simulink model "helico_model_kne24"  (R2017a)
settings: Solver=FixedStepAuto  StartTime=0.0  StopTime=par.tend  FixedStep=par.ts  MaxStep=1e-3  RelTol=1e-3
values from neighbouring files (symbols this model uses):
  N = 4001    [workspace.mat]
  par =     [workspace.mat]
  par_id = struct    [model_benchmark_init.m]    (also in workspace.mat = )
undefined symbols (not defined in the file or in its folder): X, Y, Z
libraries: sm_lib x25, nesl_utility x11, simulink x1
settings Model: Creator=mirko  LastModifiedBy=obrusvit

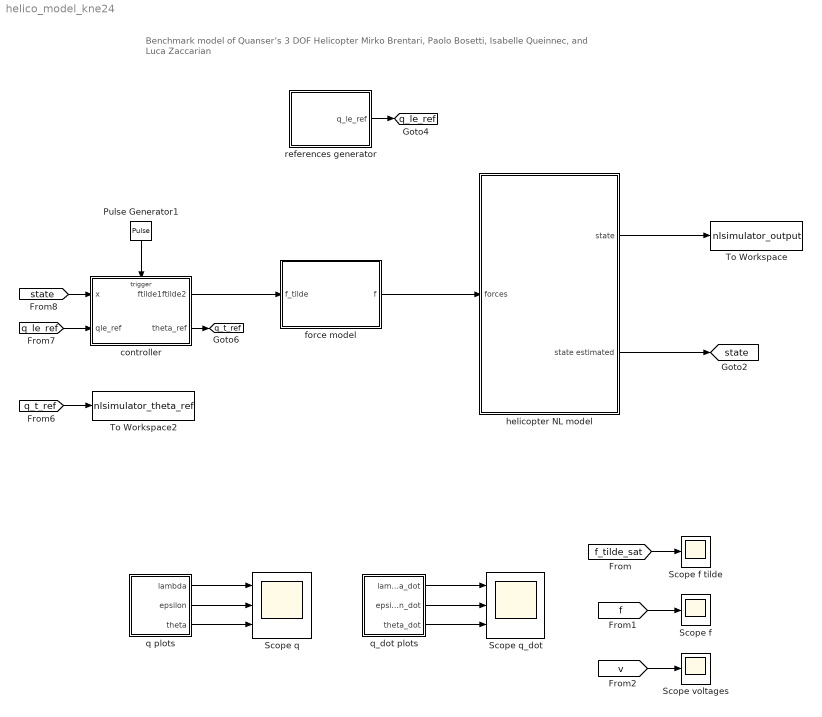
== system helico_model_kne24 ==
  note: Benchmark model of Quanser’s 3 DOF Helicopter
      | Mirko Brentari, Paolo Bosetti, Isabelle Queinnec, and Luca Zaccarian
  Pulse Generator1 : DiscretePulseGenerator  PulseType=Time based  Period=0.01  PulseWidth=50
  Scope f : Scope
  Scope f tilde : Scope
  Scope q : Scope  NumInputPorts=3
  Scope q_dot : Scope  NumInputPorts=3
  Scope voltages : Scope
  To Workspace : ToWorkspace  VariableName=nlsimulator_output  SaveFormat=Timeseries  SampleTime=-1
  To Workspace2 : ToWorkspace  VariableName=nlsimulator_theta_ref  SaveFormat=Timeseries  SampleTime=-1
  controller : Subsystem
  force model : Subsystem
  helicopter NL model : Subsystem
  q plots : Subsystem
  q_dot plots : Subsystem
  references generator : Subsystem
  tag scope: q_le_ref=global, q_t_ref=global, state=global
  wires:
  helicopter NL model/1(state) -> To Workspace/1
  references generator/1(q_le_ref) -> [q_le_ref]
  q plots/2(epsilon) -> Scope q/2
  q plots/1(lambda) -> Scope q/1
  q_dot plots/1(lambda_dot) -> Scope q_dot/1
  q plots/3(theta) -> Scope q/3
  q_dot plots/3(theta_dot) -> Scope q_dot/3
  q_dot plots/2(epsilon_dot) -> Scope q_dot/2
  helicopter NL model/2(state estimated) -> [state]
  [q_t_ref] -> To Workspace2/1
  Pulse Generator1/1 -> controller/Trigger
  controller/2(theta_ref) -> [q_t_ref]
  [state] -> controller/1(x)
  [q_le_ref] -> controller/2(qle_ref)
  controller/1(ftilde1ftilde2) -> force model/1(f_tilde)
  force model/1(f) -> helicopter NL model/1(forces)
  [f] -> Scope f/1
  [f_tilde_sat] -> Scope f tilde/1
  [v] -> Scope voltages/1

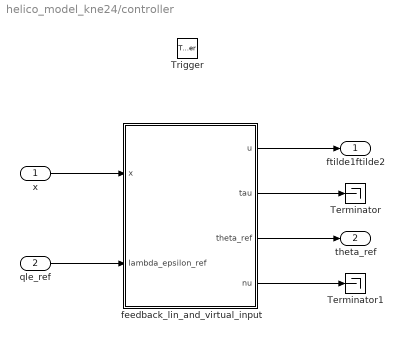
== system helico_model_kne24/controller ==
  x : Inport
  qle_ref : Inport  Port=2
  Trigger : TriggerPort  VariantControl=Variant  PortDimensions=1
  Terminator : Terminator
  Terminator1 : Terminator
  feedback_lin_and_virtual_input : MATLAB Function  TreatAsAtomicUnit=on
  ftilde1ftilde2 : Outport
  theta_ref : Outport  Port=2
  wires:
  qle_ref/1 -> feedback_lin_and_virtual_input/2(lambda_epsilon_ref)
  feedback_lin_and_virtual_input/3(theta_ref) -> theta_ref/1
  feedback_lin_and_virtual_input/2(tau) -> Terminator/1
  feedback_lin_and_virtual_input/1(u) -> ftilde1ftilde2/1
  x/1 -> feedback_lin_and_virtual_input/1(x)
  feedback_lin_and_virtual_input/4(nu) -> Terminator1/1

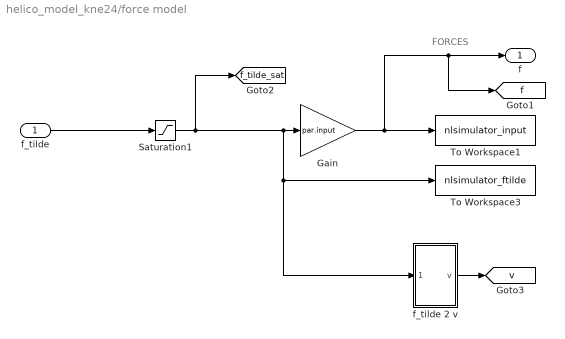
== system helico_model_kne24/force model ==
  note: FORCES
  f_tilde : Inport
  Gain : Gain  Gain=par.input
  Saturation1 : Saturate  UpperLimit=1  LowerLimit=-0.23
  To Workspace1 : ToWorkspace  VariableName=nlsimulator_input  SaveFormat=Timeseries  SampleTime=par.ts
  To Workspace3 : ToWorkspace  VariableName=nlsimulator_ftilde  SaveFormat=Timeseries  SampleTime=par.ts
  f_tilde 2 v : Subsystem
  f : Outport
  tag scope: f=global, f_tilde_sat=global, v=global
  wires:
  Saturation1/1 -> [f_tilde_sat], f_tilde 2 v/1(f_tilde), To Workspace3/1, Gain/1
  f_tilde/1 -> Saturation1/1
  Gain/1 -> [f], f/1, To Workspace1/1
  f_tilde 2 v/1(v) -> [v]

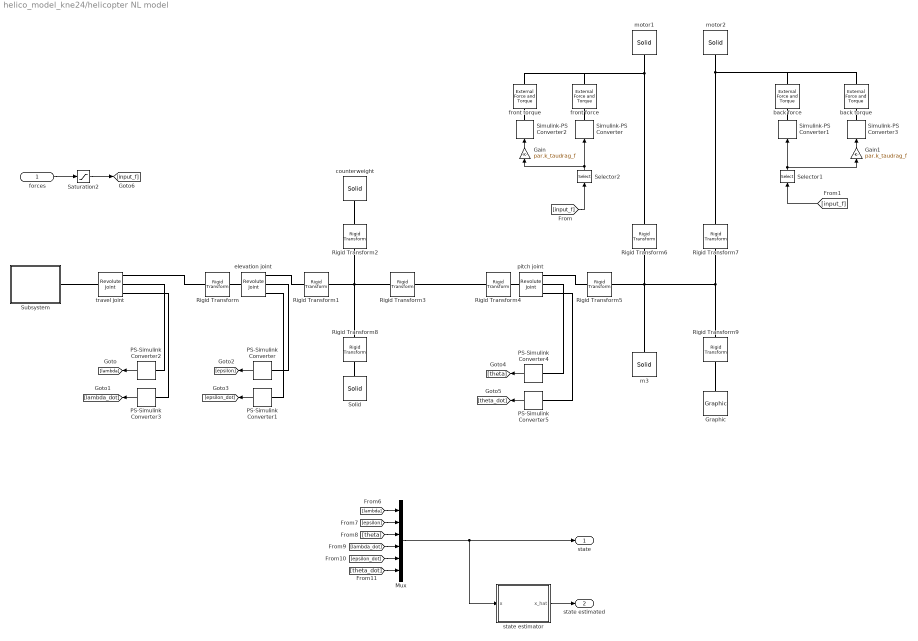
== system helico_model_kne24/helicopter NL model ==
  forces : Inport
  Gain : Gain  Gain=par.k_taudrag_f
  Gain1 : Gain  Gain=par.k_taudrag_f
  Graphic : sm_lib/Body Elements/Graphic  GraphicType=Marker  MarkerShape=Sphere  MarkerSize=10  GraphicVisPropType=SimpleVisualProperties  GraphicDiffuseColor=[1.0 0.0 0.2]  GraphicSpecularColor=[0.5 0.5 0.5 1.0]  GraphicAmbientColor=[0.15 0.15 0.15 1.0]  GraphicEmissiveColor=[0.0 0.0 0.0 1.0]  GraphicShininess=75  GraphicOpacity=0.5
      settings: SourceProductName=Simscape Multibody
  Mux : Mux  Inputs=6
  PS-Simulink Converter{,1..5} (6 alike) : nesl_utility/PS-Simulink Converter  PhysicalDomain=network_engine_domain  SubClassName=ps_output  LeftPortType=input  RightPortType=output  PseudoPeriodic=off  Frequencies=[]  Unit=1  AffineConversion=off
  Rigid Transform : sm_lib/Frames and Transforms/Rigid Transform  TranslationMethod=None  TranslationStandardOffset=0  TranslationLengthUnit=m  TranslationStandardAxis=+Z  TranslationCartesianOffset=[0 0 0]  TranslationROffset=0  TranslationROffsetUnits=m  TranslationZOffset=0  TranslationZOffsetUnits=m  TranslationThetaOffset=0  TranslationThetaOffsetUnits=deg  RotationMethod=StandardAxis  RotationAngleUnits=deg  RotationStandardAxis=+X  RotationAngle=90  RotationArbitraryAxis=[0 0 1]  FollAlignAxisA=+Z  BaseAlignAxisA=+Y  FollAlignAxisB=+X  BaseAlignAxisB=+X  RotationSequenceAxes=FollowerAxes  RotationSequence=XYX  RotationSequenceAngles=[0 0 0]  RotationSequenceAnglesUnits=deg  RotationMatrix=[1 0 0; 0 1 0; 0 0 1]
  Rigid Transform1 : sm_lib/Frames and Transforms/Rigid Transform  TranslationMethod=None  TranslationStandardOffset=0  TranslationLengthUnit=m  TranslationStandardAxis=+Z  TranslationCartesianOffset=[1 0 0]  TranslationROffset=0  TranslationROffsetUnits=m  TranslationZOffset=0  TranslationZOffsetUnits=m  TranslationThetaOffset=0  TranslationThetaOffsetUnits=deg  RotationMethod=StandardAxis  RotationAngleUnits=deg  RotationStandardAxis=+X  RotationAngle=-90  RotationArbitraryAxis=[0 0 1]  FollAlignAxisA=+Z  BaseAlignAxisA=+Y  FollAlignAxisB=+X  BaseAlignAxisB=+X  RotationSequenceAxes=FollowerAxes  RotationSequence=XYX  RotationSequenceAngles=[0 0 0]  RotationSequenceAnglesUnits=deg  RotationMatrix=[1 0 0; 0 1 0; 0 0 1]
  Rigid Transform2 : sm_lib/Frames and Transforms/Rigid Transform  TranslationMethod=Cartesian  TranslationStandardOffset=0  TranslationLengthUnit=m  TranslationStandardAxis=+Z  TranslationCartesianOffset=[-par.l1 0 -par.d1]  TranslationROffset=0  TranslationROffsetUnits=m  TranslationZOffset=0  TranslationZOffsetUnits=m  TranslationThetaOffset=0  TranslationThetaOffsetUnits=deg  RotationMethod=None  RotationAngleUnits=deg  RotationStandardAxis=+X  RotationAngle=+90  RotationArbitraryAxis=[0 0 1]  FollAlignAxisA=+Z  BaseAlignAxisA=+Y  FollAlignAxisB=+X  BaseAlignAxisB=+X  RotationSequenceAxes=FollowerAxes  RotationSequence=XYX  RotationSequenceAngles=[0 0 0]  RotationSequenceAnglesUnits=deg  RotationMatrix=[1 0 0; 0 1 0; 0 0 1]
  Rigid Transform3 : sm_lib/Frames and Transforms/Rigid Transform  TranslationMethod=Cartesian  TranslationStandardOffset=0  TranslationLengthUnit=m  TranslationStandardAxis=+Z  TranslationCartesianOffset=[par.l2 0 0]  TranslationROffset=0  TranslationROffsetUnits=m  TranslationZOffset=0  TranslationZOffsetUnits=m  TranslationThetaOffset=0  TranslationThetaOffsetUnits=deg  RotationMethod=None  RotationAngleUnits=deg  RotationStandardAxis=+X  RotationAngle=+90  RotationArbitraryAxis=[0 0 1]  FollAlignAxisA=+Z  BaseAlignAxisA=+Y  FollAlignAxisB=+X  BaseAlignAxisB=+X  RotationSequenceAxes=FollowerAxes  RotationSequence=XYX  RotationSequenceAngles=[0 0 0]  RotationSequenceAnglesUnits=deg  RotationMatrix=[1 0 0; 0 1 0; 0 0 1]
  Rigid Transform4 : sm_lib/Frames and Transforms/Rigid Transform  TranslationMethod=None  TranslationStandardOffset=0  TranslationLengthUnit=m  TranslationStandardAxis=+Z  TranslationCartesianOffset=[0 0 0]  TranslationROffset=0  TranslationROffsetUnits=m  TranslationZOffset=0  TranslationZOffsetUnits=m  TranslationThetaOffset=0  TranslationThetaOffsetUnits=deg  RotationMethod=StandardAxis  RotationAngleUnits=deg  RotationStandardAxis=+Y  RotationAngle=90  RotationArbitraryAxis=[0 0 1]  FollAlignAxisA=+Z  BaseAlignAxisA=+Y  FollAlignAxisB=+X  BaseAlignAxisB=+X  RotationSequenceAxes=FollowerAxes  RotationSequence=XYX  RotationSequenceAngles=[0 0 0]  RotationSequenceAnglesUnits=deg  RotationMatrix=[1 0 0; 0 1 0; 0 0 1]
  Rigid Transform5 : sm_lib/Frames and Transforms/Rigid Transform  TranslationMethod=None  TranslationStandardOffset=0  TranslationLengthUnit=m  TranslationStandardAxis=+Z  TranslationCartesianOffset=[1 0 0]  TranslationROffset=0  TranslationROffsetUnits=m  TranslationZOffset=0  TranslationZOffsetUnits=m  TranslationThetaOffset=0  TranslationThetaOffsetUnits=deg  RotationMethod=StandardAxis  RotationAngleUnits=deg  RotationStandardAxis=+Y  RotationAngle=-90  RotationArbitraryAxis=[0 0 1]  FollAlignAxisA=+Z  BaseAlignAxisA=+Y  FollAlignAxisB=+X  BaseAlignAxisB=+X  RotationSequenceAxes=FollowerAxes  RotationSequence=XYX  RotationSequenceAngles=[0 0 0]  RotationSequenceAnglesUnits=deg  RotationMatrix=[1 0 0; 0 1 0; 0 0 1]
  Rigid Transform6 : sm_lib/Frames and Transforms/Rigid Transform  TranslationMethod=Cartesian  TranslationStandardOffset=0  TranslationLengthUnit=m  TranslationStandardAxis=+Z  TranslationCartesianOffset=[0 par.l3 -par.d2]  TranslationROffset=0  TranslationROffsetUnits=m  TranslationZOffset=0  TranslationZOffsetUnits=m  TranslationThetaOffset=0  TranslationThetaOffsetUnits=deg  RotationMethod=None  RotationAngleUnits=deg  RotationStandardAxis=+X  RotationAngle=+90  RotationArbitraryAxis=[0 0 1]  FollAlignAxisA=+Z  BaseAlignAxisA=+Y  FollAlignAxisB=+X  BaseAlignAxisB=+X  RotationSequenceAxes=FollowerAxes  RotationSequence=XYX  RotationSequenceAngles=[0 0 0]  RotationSequenceAnglesUnits=deg  RotationMatrix=[1 0 0; 0 1 0; 0 0 1]
  Rigid Transform7 : sm_lib/Frames and Transforms/Rigid Transform  TranslationMethod=Cartesian  TranslationStandardOffset=0  TranslationLengthUnit=m  TranslationStandardAxis=+Z  TranslationCartesianOffset=[0 -par.l3 -par.d2]  TranslationROffset=0  TranslationROffsetUnits=m  TranslationZOffset=0  TranslationZOffsetUnits=m  TranslationThetaOffset=0  TranslationThetaOffsetUnits=deg  RotationMethod=None  RotationAngleUnits=deg  RotationStandardAxis=+X  RotationAngle=+90  RotationArbitraryAxis=[0 0 1]  FollAlignAxisA=+Z  BaseAlignAxisA=+Y  FollAlignAxisB=+X  BaseAlignAxisB=+X  RotationSequenceAxes=FollowerAxes  RotationSequence=XYX  RotationSequenceAngles=[0 0 0]  RotationSequenceAnglesUnits=deg  RotationMatrix=[1 0 0; 0 1 0; 0 0 1]
  Rigid Transform8 : sm_lib/Frames and Transforms/Rigid Transform  TranslationMethod=Cartesian  TranslationStandardOffset=0  TranslationLengthUnit=m  TranslationStandardAxis=+Z  TranslationCartesianOffset=[(par.l1+par.l2)/2-par.l1 0 0]  TranslationROffset=0  TranslationROffsetUnits=m  TranslationZOffset=0  TranslationZOffsetUnits=m  TranslationThetaOffset=0  TranslationThetaOffsetUnits=deg  RotationMethod=AlignedAxes  RotationAngleUnits=deg  RotationStandardAxis=+X  RotationAngle=+90  RotationArbitraryAxis=[0 0 1]  FollAlignAxisA=+Z  BaseAlignAxisA=+X  FollAlignAxisB=+Y  BaseAlignAxisB=+Y  RotationSequenceAxes=FollowerAxes  RotationSequence=XYX  RotationSequenceAngles=[0 0 0]  RotationSequenceAnglesUnits=deg  RotationMatrix=[1 0 0; 0 1 0; 0 0 1]
  Rigid Transform9 : sm_lib/Frames and Transforms/Rigid Transform  TranslationMethod=Cartesian  TranslationStandardOffset=0  TranslationLengthUnit=m  TranslationStandardAxis=+Z  TranslationCartesianOffset=[0 0 -par.d2]  TranslationROffset=0  TranslationROffsetUnits=m  TranslationZOffset=0  TranslationZOffsetUnits=m  TranslationThetaOffset=0  TranslationThetaOffsetUnits=deg  RotationMethod=None  RotationAngleUnits=deg  RotationStandardAxis=+X  RotationAngle=+90  RotationArbitraryAxis=[0 0 1]  FollAlignAxisA=+Z  BaseAlignAxisA=+X  FollAlignAxisB=+Y  BaseAlignAxisB=+Y  RotationSequenceAxes=FollowerAxes  RotationSequence=XYX  RotationSequenceAngles=[0 0 0]  RotationSequenceAnglesUnits=deg  RotationMatrix=[1 0 0; 0 1 0; 0 0 1]
  Saturation2 : Saturate  UpperLimit=1*par.input  LowerLimit=-0.23*par.input
  Selector1 : Selector  InputPortWidth=2  IndexOptions=Index vector (dialog)  Indices=2  OutputSizes=1
  Selector2 : Selector  InputPortWidth=2  IndexOptions=Index vector (dialog)  Indices=1  OutputSizes=1
  Simulink-PS Converter{,1..3} (4 alike) : nesl_utility/Simulink-PS Converter  PhysicalDomain=network_engine_domain  SubClassName=ps_input  LeftPortType=input  RightPortType=output  PseudoPeriodic=off  Frequencies=[]  NoiseDistribution=none  NoiseParameters=[]  Unit=1  AffineConversion=off  FilteringAndDerivatives=provide  SimscapeFilterOrder=1  InputFilterTimeConstant=0.001  UdotUserProvided=0
  Solid : sm_lib/Body Elements/Solid  InertiaType=CalculateFromGeometry  Mass=1  MassUnits=kg  CenterOfMass=[0 0 0]  CenterOfMassUnits=m  MomentsOfInertia=[1 1 1]  MomentsOfInertiaUnits=kg*m^2  ProductsOfInertia=[1 1 1]  ProductsOfInertiaUnits=kg*m^2  DensityBased=on  Density=0  DensityUnits=kg/m^3  DoExposeReferenceFrame=on  SerializedFrames=<Frames/>  GraphicType=FromGeometry  MarkerShape=Sphere  MarkerSize=10  GraphicVisPropType=SimpleVisualProperties  GraphicDiffuseColor=[0.5 0.5 0.5]  GraphicSpecularColor=[0.5 0.5 0.5 1.0]  GraphicAmbientColor=[0.15 0.15 0.15 1.0]  GraphicEmissiveColor=[0.0 0.0 0.0 1.0]  GraphicShininess=75  GraphicOpacity=0.5  GeometryShape=Cylinder  RectangleSize=[1 1]  RectangleSizeUnits=m  BrickDimensions=[1 1 1]  BrickDimensionUnits=m  CylinderRadius=0.005  CylinderRadiusUnits=m  CylinderLength=par.l1+par.l2  CylinderLengthUnits=m  SphereRadius=1  SphereRadiusUnits=m  EllipsoidRadii=[1 1 1]  EllipsoidRadiiUnits=m  ExtrusionCrossSection=[1 1; -1 1; -1 -1; 1 -1]  ExtrusionCrossSectionUnits=m  ExtrusionLength=1  ExtrusionLengthUnits=m  PolygonNumSides=3  PolygonOuterRadius=1  PolygonOuterRadiusUnits=m  ExtGeomFileType=STEP  ExtGeomFileUnits=m  RevolutionCrossSection=[1 1; 1 -1; 2 -1; 2 1]  RevolutionCrossSectionUnits=m  RevolutionExtent=Full  RevolutionAngle=180  RevolutionAngleUnits=deg
  Subsystem : Subsystem
  back force : sm_lib/Forces and Torques/External Force and Torque  ForceResolutionFrame=AttachedFrame  EnableForceX=off  EnableForceY=off  EnableForceZ=on  EnableForce=off  TorqueResolutionFrame=AttachedFrame  EnableTorqueX=off  EnableTorqueY=off  EnableTorqueZ=off  EnableTorque=off
  back torque : sm_lib/Forces and Torques/External Force and Torque  ForceResolutionFrame=AttachedFrame  EnableForceX=off  EnableForceY=off  EnableForceZ=off  EnableForce=off  TorqueResolutionFrame=AttachedFrame  EnableTorqueX=off  EnableTorqueY=off  EnableTorqueZ=on  EnableTorque=off
  counterweight : sm_lib/Body Elements/Solid  InertiaType=PointMass  Mass=par.m1  MassUnits=kg  CenterOfMass=[0 0 0]  CenterOfMassUnits=m  MomentsOfInertia=[1 1 1]  MomentsOfInertiaUnits=kg*m^2  ProductsOfInertia=[1 1 1]  ProductsOfInertiaUnits=kg*m^2  DensityBased=on  Density=1000  DensityUnits=kg/m^3  DoExposeReferenceFrame=on  SerializedFrames=<Frames/>  GraphicType=FromGeometry  MarkerShape=Sphere  MarkerSize=10  GraphicVisPropType=AdvancedVisualProperties  GraphicDiffuseColor=[0.5 0.5 0.5]  GraphicSpecularColor=[0.5 0.5 0.5 1.0]  GraphicAmbientColor=[0.15 0.15 0.15 1.0]  GraphicEmissiveColor=[0.0 0.0 0.0 1.0]  GraphicShininess=75  GraphicOpacity=1.0  GeometryShape=Sphere  RectangleSize=[1 1]  RectangleSizeUnits=m  BrickDimensions=[1 1 1]  BrickDimensionUnits=m  CylinderRadius=1  CylinderRadiusUnits=m  CylinderLength=1  CylinderLengthUnits=m  SphereRadius=0.1  SphereRadiusUnits=m  EllipsoidRadii=[1 1 1]  EllipsoidRadiiUnits=m  ExtrusionCrossSection=[1 1; -1 1; -1 -1; 1 -1]  ExtrusionCrossSectionUnits=m  ExtrusionLength=1  ExtrusionLengthUnits=m  PolygonNumSides=3  PolygonOuterRadius=1  PolygonOuterRadiusUnits=m  ExtGeomFileType=STEP  ExtGeomFileUnits=m  RevolutionCrossSection=[1 1; 1 -1; 2 -1; 2 1]  RevolutionCrossSectionUnits=m  RevolutionExtent=Full  RevolutionAngle=180  RevolutionAngleUnits=deg
  elevation joint : sm_lib/Joints/Revolute Joint  SenseConstraintForce=off  SenseConstraintForceX=off  SenseConstraintForceY=off  SenseConstraintForceZ=off  SenseConstraintTorque=off  SenseConstraintTorqueX=off  SenseConstraintTorqueY=off  SenseConstraintTorqueZ=off  SenseTotalForce=off  SenseTotalForceX=off  SenseTotalForceY=off  SenseTotalForceZ=off  SenseTotalTorque=off  SenseTotalTorqueX=off  SenseTotalTorqueY=off  SenseTotalTorqueZ=off  CompositeWrenchDir=FollowerOnBase  CompositeWrenchFrame=BaseFrame  EquilibriumPosition=par.epsilon_0 * par.lock_epsilon  EquilibriumPositionUnits=rad  SpringStiffness=par.k_lock * par.lock_epsilon  SpringStiffnessUnits=N*m/rad  DampingCoefficient=par.r_epsilon  DampingCoefficientUnits=N*m/(rad/s)  TorqueActuationMode=NoTorque  MotionActuationMode=ComputedMotion  SensePosition=on  SenseVelocity=on  SenseAcceleration=off  SenseTorqueForce=off  PositionTargetSpecify=on  PositionTargetPriority=High  PositionTargetValue=par.epsilon_0  PositionTargetValueUnits=rad  VelocityTargetSpecify=off  VelocityTargetPriority=High  VelocityTargetValue=0  VelocityTargetValueUnits=deg/s
  front force : sm_lib/Forces and Torques/External Force and Torque  ForceResolutionFrame=AttachedFrame  EnableForceX=off  EnableForceY=off  EnableForceZ=on  EnableForce=off  TorqueResolutionFrame=AttachedFrame  EnableTorqueX=off  EnableTorqueY=off  EnableTorqueZ=off  EnableTorque=off
  front torque : sm_lib/Forces and Torques/External Force and Torque  ForceResolutionFrame=AttachedFrame  EnableForceX=off  EnableForceY=off  EnableForceZ=off  EnableForce=off  TorqueResolutionFrame=AttachedFrame  EnableTorqueX=off  EnableTorqueY=off  EnableTorqueZ=on  EnableTorque=off
  m3 : sm_lib/Body Elements/Solid  InertiaType=PointMass  Mass=par.m3  MassUnits=kg  CenterOfMass=[0 0 0]  CenterOfMassUnits=m  MomentsOfInertia=[1 1 1]  MomentsOfInertiaUnits=kg*m^2  ProductsOfInertia=[1 1 1]  ProductsOfInertiaUnits=kg*m^2  DensityBased=on  Density=1000  DensityUnits=kg/m^3  DoExposeReferenceFrame=on  SerializedFrames=<Frames/>  GraphicType=FromGeometry  MarkerShape=Sphere  MarkerSize=10  GraphicVisPropType=SimpleVisualProperties  GraphicDiffuseColor=[0.0 0.6 0.0]  GraphicSpecularColor=[0.5 0.5 0.5 1.0]  GraphicAmbientColor=[0.15 0.15 0.15 1.0]  GraphicEmissiveColor=[0.0 0.0 0.0 1.0]  GraphicShininess=75  GraphicOpacity=1.0  GeometryShape=Sphere  RectangleSize=[1 1]  RectangleSizeUnits=m  BrickDimensions=[1 1 1]  BrickDimensionUnits=m  CylinderRadius=0.05  CylinderRadiusUnits=m  CylinderLength=0.05  CylinderLengthUnits=m  SphereRadius=0.01  SphereRadiusUnits=m  EllipsoidRadii=[1 1 1]  EllipsoidRadiiUnits=m  ExtrusionCrossSection=[1 1; -1 1; -1 -1; 1 -1]  ExtrusionCrossSectionUnits=m  ExtrusionLength=1  ExtrusionLengthUnits=m  PolygonNumSides=3  PolygonOuterRadius=1  PolygonOuterRadiusUnits=m  ExtGeomFileType=STEP  ExtGeomFileUnits=m  RevolutionCrossSection=[1 1; 1 -1; 2 -1; 2 1]  RevolutionCrossSectionUnits=m  RevolutionExtent=Full  RevolutionAngle=180  RevolutionAngleUnits=deg
  motor1 : sm_lib/Body Elements/Solid  InertiaType=PointMass  Mass=par.m2/2  MassUnits=kg  CenterOfMass=[0 0 0]  CenterOfMassUnits=m  MomentsOfInertia=[1 1 1]  MomentsOfInertiaUnits=kg*m^2  ProductsOfInertia=[1 1 1]  ProductsOfInertiaUnits=kg*m^2  DensityBased=on  Density=1000  DensityUnits=kg/m^3  DoExposeReferenceFrame=on  SerializedFrames=<Frames/>  GraphicType=FromGeometry  MarkerShape=Sphere  MarkerSize=10  GraphicVisPropType=SimpleVisualProperties  GraphicDiffuseColor=[0.4 0.4 0.5019608]  GraphicSpecularColor=[0.5 0.5 0.5 1.0]  GraphicAmbientColor=[0.15 0.15 0.15 1.0]  GraphicEmissiveColor=[0.0 0.0 0.0 1.0]  GraphicShininess=75  GraphicOpacity=1.0  GeometryShape=Cylinder  RectangleSize=[1 1]  RectangleSizeUnits=m  BrickDimensions=[1 1 1]  BrickDimensionUnits=m  CylinderRadius=0.05  CylinderRadiusUnits=m  CylinderLength=0.05  CylinderLengthUnits=m  SphereRadius=0.1  SphereRadiusUnits=m  EllipsoidRadii=[1 1 1]  EllipsoidRadiiUnits=m  ExtrusionCrossSection=[1 1; -1 1; -1 -1; 1 -1]  ExtrusionCrossSectionUnits=m  ExtrusionLength=1  ExtrusionLengthUnits=m  PolygonNumSides=3  PolygonOuterRadius=1  PolygonOuterRadiusUnits=m  ExtGeomFileType=STEP  ExtGeomFileUnits=m  RevolutionCrossSection=[1 1; 1 -1; 2 -1; 2 1]  RevolutionCrossSectionUnits=m  RevolutionExtent=Full  RevolutionAngle=180  RevolutionAngleUnits=deg
  motor2 : sm_lib/Body Elements/Solid  InertiaType=PointMass  Mass=par.m2/2  MassUnits=kg  CenterOfMass=[0 0 0]  CenterOfMassUnits=m  MomentsOfInertia=[1 1 1]  MomentsOfInertiaUnits=kg*m^2  ProductsOfInertia=[1 1 1]  ProductsOfInertiaUnits=kg*m^2  DensityBased=on  Density=1000  DensityUnits=kg/m^3  DoExposeReferenceFrame=on  SerializedFrames=<Frames/>  GraphicType=FromGeometry  MarkerShape=Sphere  MarkerSize=10  GraphicVisPropType=SimpleVisualProperties  GraphicDiffuseColor=[0.49803922 0.4 0.4]  GraphicSpecularColor=[0.5 0.5 0.5 1.0]  GraphicAmbientColor=[0.15 0.15 0.15 1.0]  GraphicEmissiveColor=[0.0 0.0 0.0 1.0]  GraphicShininess=75  GraphicOpacity=1.0  GeometryShape=Cylinder  RectangleSize=[1 1]  RectangleSizeUnits=m  BrickDimensions=[1 1 1]  BrickDimensionUnits=m  CylinderRadius=0.05  CylinderRadiusUnits=m  CylinderLength=0.05  CylinderLengthUnits=m  SphereRadius=0.1  SphereRadiusUnits=m  EllipsoidRadii=[1 1 1]  EllipsoidRadiiUnits=m  ExtrusionCrossSection=[1 1; -1 1; -1 -1; 1 -1]  ExtrusionCrossSectionUnits=m  ExtrusionLength=1  ExtrusionLengthUnits=m  PolygonNumSides=3  PolygonOuterRadius=1  PolygonOuterRadiusUnits=m  ExtGeomFileType=STEP  ExtGeomFileUnits=m  RevolutionCrossSection=[1 1; 1 -1; 2 -1; 2 1]  RevolutionCrossSectionUnits=m  RevolutionExtent=Full  RevolutionAngle=180  RevolutionAngleUnits=deg
  pitch joint : sm_lib/Joints/Revolute Joint  SenseConstraintForce=off  SenseConstraintForceX=off  SenseConstraintForceY=off  SenseConstraintForceZ=off  SenseConstraintTorque=off  SenseConstraintTorqueX=off  SenseConstraintTorqueY=off  SenseConstraintTorqueZ=off  SenseTotalForce=off  SenseTotalForceX=off  SenseTotalForceY=off  SenseTotalForceZ=off  SenseTotalTorque=off  SenseTotalTorqueX=off  SenseTotalTorqueY=off  SenseTotalTorqueZ=off  CompositeWrenchDir=FollowerOnBase  CompositeWrenchFrame=BaseFrame  EquilibriumPosition=par.theta_0 * par.lock_theta  EquilibriumPositionUnits=rad  SpringStiffness=par.k_lock * par.lock_theta  SpringStiffnessUnits=N*m/rad  DampingCoefficient=par.r_theta  DampingCoefficientUnits=N*m/(rad/s)  TorqueActuationMode=NoTorque  MotionActuationMode=ComputedMotion  SensePosition=on  SenseVelocity=on  SenseAcceleration=off  SenseTorqueForce=off  PositionTargetSpecify=on  PositionTargetPriority=High  PositionTargetValue=par.theta_0  PositionTargetValueUnits=rad  VelocityTargetSpecify=on  VelocityTargetPriority=High  VelocityTargetValue=par.theta_dot_0  VelocityTargetValueUnits=rad/s
  state estimator : Subsystem
  travel joint : sm_lib/Joints/Revolute Joint  SenseConstraintForce=off  SenseConstraintForceX=off  SenseConstraintForceY=off  SenseConstraintForceZ=off  SenseConstraintTorque=off  SenseConstraintTorqueX=off  SenseConstraintTorqueY=off  SenseConstraintTorqueZ=off  SenseTotalForce=off  SenseTotalForceX=off  SenseTotalForceY=off  SenseTotalForceZ=off  SenseTotalTorque=off  SenseTotalTorqueX=off  SenseTotalTorqueY=off  SenseTotalTorqueZ=off  CompositeWrenchDir=FollowerOnBase  CompositeWrenchFrame=BaseFrame  EquilibriumPosition=par.lambda_0 * par.lock_lambda  EquilibriumPositionUnits=rad  SpringStiffness=par.k_lock * par.lock_lambda  SpringStiffnessUnits=N*m/rad  DampingCoefficient=par.r_lambda  DampingCoefficientUnits=N*m/(rad/s)  TorqueActuationMode=NoTorque  MotionActuationMode=ComputedMotion  SensePosition=on  SenseVelocity=on  SenseAcceleration=off  SenseTorqueForce=off  PositionTargetSpecify=on  PositionTargetPriority=High  PositionTargetValue=par.lambda_0  PositionTargetValueUnits=rad  VelocityTargetSpecify=off  VelocityTargetPriority=High  VelocityTargetValue=0  VelocityTargetValueUnits=deg/s
  state : Outport
  state estimated : Outport  Port=2
  wires:
  [lambda] -> Mux/1
  [epsilon] -> Mux/2
  PS-Simulink Converter/1 -> [epsilon]
  PS-Simulink Converter1/1 -> [epsilon_dot]
  PS-Simulink Converter3/1 -> [lambda_dot]
  PS-Simulink Converter2/1 -> [lambda]
  PS-Simulink Converter5/1 -> [theta_dot]
  PS-Simulink Converter4/1 -> [theta]
  [theta] -> Mux/3
  [theta_dot] -> Mux/6
  Mux/1 -> state estimator/1(x), state/1
  [epsilon_dot] -> Mux/5
  [lambda_dot] -> Mux/4
  [input_f] -> Selector1/1
  state estimator/1(x_hat) -> state estimated/1
  Gain/1 -> Simulink-PS Converter2/1
  [input_f] -> Selector2/1
  Selector2/1 -> Gain/1, Simulink-PS Converter/1
  Selector1/1 -> Gain1/1, Simulink-PS Converter1/1
  Gain1/1 -> Simulink-PS Converter3/1
  forces/1 -> Saturation2/1
  Saturation2/1 -> [input_f]
  connections:
  Rigid Transform/RConn1 -- elevation joint/LConn1
  Rigid Transform5/LConn1 -- pitch joint/RConn1
  travel joint/RConn1 -- Rigid Transform/LConn1
  Rigid Transform4/RConn1 -- pitch joint/LConn1
  Rigid Transform3/RConn1 -- Rigid Transform4/LConn1
  Rigid Transform2/LConn1 -- Rigid Transform3/LConn1 -- Rigid Transform1/RConn1 -- Rigid Transform8/LConn1
  Rigid Transform8/RConn1 -- Solid/RConn1
  PS-Simulink Converter/LConn1 -- elevation joint/RConn2
  Rigid Transform1/LConn1 -- elevation joint/RConn1
  PS-Simulink Converter1/LConn1 -- elevation joint/RConn3
  PS-Simulink Converter2/LConn1 -- travel joint/RConn2
  PS-Simulink Converter3/LConn1 -- travel joint/RConn3
  PS-Simulink Converter4/LConn1 -- pitch joint/RConn2
  PS-Simulink Converter5/LConn1 -- pitch joint/RConn3
  motor1/RConn1 -- front torque/RConn1 -- front force/RConn1 -- Rigid Transform6/RConn1
  counterweight/RConn1 -- Rigid Transform2/RConn1
  motor2/RConn1 -- back torque/RConn1 -- back force/RConn1 -- Rigid Transform7/RConn1
  Rigid Transform5/RConn1 -- m3/RConn1 -- Rigid Transform6/LConn1 -- Rigid Transform9/LConn1 -- Rigid Transform7/LConn1
  Graphic/RConn1 -- Rigid Transform9/RConn1
  Subsystem/RConn1 -- travel joint/LConn1
  Simulink-PS Converter1/RConn1 -- back force/LConn1
  Simulink-PS Converter/RConn1 -- front force/LConn1
  Simulink-PS Converter2/RConn1 -- front torque/LConn1
  Simulink-PS Converter3/RConn1 -- back torque/LConn1

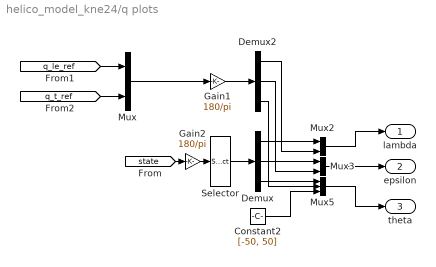
== system helico_model_kne24/q plots ==
  Constant2 : Constant  Value=[-50, 50]
  Demux : Demux  Outputs=3
  Demux2 : Demux  Outputs=3
  Gain1 : Gain  Gain=180/pi
  Gain2 : Gain  Gain=180/pi
  Mux : Mux  Inputs=2
  Mux2 : Mux  Inputs=2
  Mux3 : Mux  Inputs=2
  Mux5 : Mux  Inputs=3
  Selector : Selector  InputPortWidth=6  IndexOptions=Index vector (dialog)  Indices=1:3  OutputSizes=1
  lambda : Outport
  epsilon : Outport  Port=2
  theta : Outport  Port=3
  wires:
  Constant2/1 -> Mux5/3
  Mux5/1 -> theta/1
  Demux/2 -> Mux3/1
  Mux3/1 -> epsilon/1
  Mux2/1 -> lambda/1
  Gain1/1 -> Demux2/1
  Demux2/1 -> Mux2/2
  Demux2/2 -> Mux3/2
  Gain2/1 -> Selector/1
  Mux/1 -> Gain1/1
  Demux2/3 -> Mux5/2
  Selector/1 -> Demux/1
  Demux/1 -> Mux2/1
  [state] -> Gain2/1
  Demux/3 -> Mux5/1
  [q_t_ref] -> Mux/2
  [q_le_ref] -> Mux/1

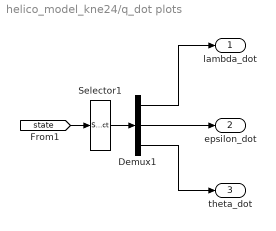
== system helico_model_kne24/q_dot plots ==
  Demux1 : Demux  Outputs=3
  Selector1 : Selector  InputPortWidth=6  IndexOptions=Index vector (dialog)  Indices=4:6  OutputSizes=1
  lambda_dot : Outport
  epsilon_dot : Outport  Port=2
  theta_dot : Outport  Port=3
  wires:
  [state] -> Selector1/1
  Demux1/1 -> lambda_dot/1
  Demux1/3 -> theta_dot/1
  Demux1/2 -> epsilon_dot/1
  Selector1/1 -> Demux1/1

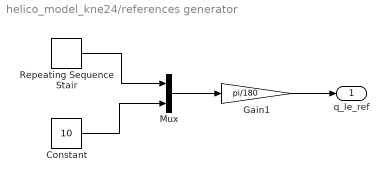
== system helico_model_kne24/references generator ==
  Constant : Constant  Value=10
  Gain1 : Gain  Gain=pi/180
  Mux : Mux  Inputs=2
  Repeating Sequence Stair : simulink/Sources/Repeating Sequence Stair  OutValues=[0 90 0 -90].'  tsamp=10  OutMin=[]  OutMax=[]  OutDataTypeStr=double  OutputDataTypeScalingMode=double  OutDataType=fixdt(0,8)  ConRadixGroup=Best Precision: Vector-wise  OutScaling=2^-12
  q_le_ref : Outport
  wires:
  Gain1/1 -> q_le_ref/1
  Mux/1 -> Gain1/1
  Repeating Sequence Stair/1 -> Mux/1
  Constant/1 -> Mux/2

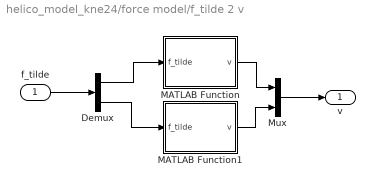
== system helico_model_kne24/force model/f_tilde 2 v ==
  f_tilde : Inport
  Demux : Demux  Outputs=2
  MATLAB Function : MATLAB Function  TreatAsAtomicUnit=on
  MATLAB Function1 : MATLAB Function  TreatAsAtomicUnit=on
  Mux : Mux  Inputs=2
  v : Outport
  wires:
  MATLAB Function/1(v) -> Mux/1
  f_tilde/1 -> Demux/1
  Demux/2 -> MATLAB Function1/1(f_tilde)
  Mux/1 -> v/1
  MATLAB Function1/1(v) -> Mux/2
  Demux/1 -> MATLAB Function/1(f_tilde)

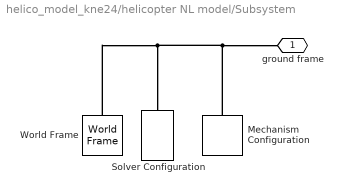
== system helico_model_kne24/helicopter NL model/Subsystem ==
  Mechanism Configuration : sm_lib/Utilities/Mechanism Configuration  UniformGravity=Constant  GravityVector=[0 0 -par.g]  GravityUnits=m/s^2  LinearizationDelta=0.001
  Solver Configuration : nesl_utility/Solver Configuration  PhysicalDomain=network_engine_domain  SubClassName=solver  LeftPortType=input  RightPortType=generic  Accelerate=off  Tones=[]  Harmonics=[]  SimulateNoise=off  Profile=off  UseLocalSampling=off  EnableSwitchedLinearOptims=on  FrequencyDomain=off  UseCCode=off  RelTol=0.001  AbsTol=1e-06  MinStep=1e-09  ToWorkspace=off  RevertToSquareIcSolve=off  NumHomotopyIterations=100  PhasorMode=off  PhasorModeNumHarmonics=1  OverrideAbsTol=off  DoDC=off  ResidualTolerance=1e-09  UseLocalSolver=off  LocalSolverChoice=NE_BACKWARD_EULER_ADVANCER  LocalSolverSampleTime=0.001  DoFixedCost=off  MaxNonlinIter=3  MaxModeIter=2  LinearAlgebra=Sparse  DelaysMemoryBudget=1024  AutomaticFiltering=on  FilteringTimeConstant=0.001
  World Frame : sm_lib/Frames and Transforms/World Frame
  ground frame : PMIOPort  Port=1  Side=Right
  connections:
  Mechanism Configuration/RConn1 -- ground frame/RConn1 -- World Frame/RConn1 -- Solver Configuration/RConn1

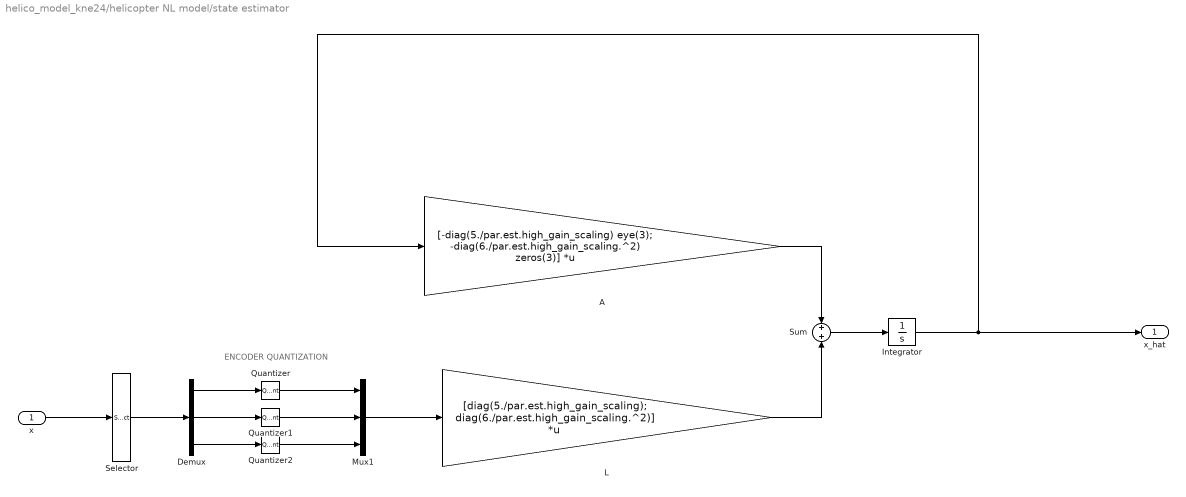
== system helico_model_kne24/helicopter NL model/state estimator ==
  note: ENCODER QUANTIZATION
  x : Inport
  A : Gain  Gain=[-diag(5./par.est.high_gain_scaling) eye(3); -diag(6./par.est.high_gain_scaling.^2) zeros(3)]  Multiplication=Matrix(K*u)
  Demux : Demux  Outputs=3
  Integrator : Integrator  InitialCondition=[par.lambda_0; par.epsilon_0; par.theta_0; 0; 0; 0]
  L : Gain  Gain=[diag(5./par.est.high_gain_scaling); diag(6./par.est.high_gain_scaling.^2)]  Multiplication=Matrix(K*u)
  Mux1 : Mux  Inputs=3
  Quantizer : Quantizer  QuantizationInterval=0.0015
  Quantizer1 : Quantizer  QuantizationInterval=0.0015
  Quantizer2 : Quantizer  QuantizationInterval=0.0015
  Selector : Selector  InputPortWidth=6  IndexOptions=Index vector (dialog)  Indices=1:3  OutputSizes=1
  Sum : Sum
  x_hat : Outport
  wires:
  A/1 -> Sum/1
  L/1 -> Sum/2
  Sum/1 -> Integrator/1
  Mux1/1 -> L/1
  Demux/1 -> Quantizer/1
  Demux/2 -> Quantizer1/1
  Demux/3 -> Quantizer2/1
  Selector/1 -> Demux/1
  x/1 -> Selector/1
  Quantizer/1 -> Mux1/1
  Quantizer1/1 -> Mux1/2
  Quantizer2/1 -> Mux1/3
  Integrator/1 -> x_hat/1, A/1

== matlab function helico_model_kne24/force model/f_tilde 2 v/MATLAB Function ==
  data: f_tilde input; v output; par parameter
function v = fcn(f_tilde, par)

v = scaled_force_2_voltage( f_tilde, par.exp.scaled_f_2_v_par, par.exp.scaled_f_2_v_ths );

== matlab function helico_model_kne24/force model/f_tilde 2 v/MATLAB Function1 ==
  data: f_tilde input; v output; par parameter
function v = fcn(f_tilde, par)

v = scaled_force_2_voltage( f_tilde, par.exp.scaled_f_2_v_par, par.exp.scaled_f_2_v_ths );

== matlab function helico_model_kne24/controller/feedback_lin_and_virtual_input ==
  data: x input; lambda_epsilon_ref input; u output; par_id parameter; tau output; theta_ref output; nu output; par parameter
function [u, tau, theta_ref, nu] = fcn(x, lambda_epsilon_ref, par_id, par)

T = diag([-par_id.bl*cos(x(2)), par_id.be, par_id.bt]);

g_bar = [0;...
         sin(x(2))*(par_id.ae1+par_id.ae2*cos(x(3)))*0.95;...
         par_id.at*cos(x(2))*sin(x(3))];

R_bar = diag([par_id.cl, par_id.ce, par_id.ct]);
                    

nu = [0;0;0];

nu(1:2) = pinv(T(1:2, 1:2)) * ( g_bar(1:2)   -   par.ctrl.Omega(1:2,1:2)^2 * (x(1:2)-lambda_epsilon_ref)   +   (R_bar(1:2,1:2) - par.ctrl.Xi(1:2,1:2)) * x(4:5) );
nu(1) = nu(1) - 0.12;

theta_ref = atan2( nu(1), nu(2) );

if abs(x(2)<deg2rad(1))
    theta_ref = 0;
end


nu(3)   = pinv(T(3, 3)) * (g_bar(3)   -   par.ctrl.Omega(3,3)^2 * (x(3)-theta_ref)   +   (R_bar(3,3) - par.ctrl.Xi(3,3)) * x(6));

B = [sin(x(3)) 0;...
      cos(x(3)) 0;...
     0          1];
tau = B'*nu;

u = [1/2  1/2;...
     1/2 -1/2]* tau;
